simulink model "simulazionesimulinkprogetto"  (R2021a)
settings: Solver=VariableStepAuto  StartTime=0.0  StopTime=10.0  RelTol=1e-3
undefined symbols (not defined in the file): A, B, C, D
libraries: simulink x1
settings Model: Creator=micha  LastModifiedBy=micha

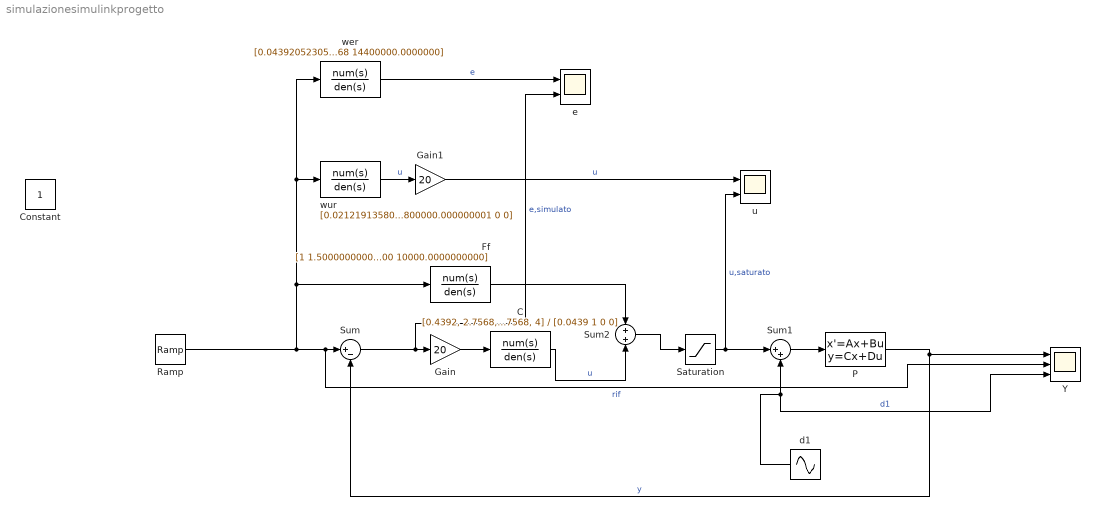
== system simulazionesimulinkprogetto ==
  C : TransferFcn  Numerator=[0.4392, 2.7568, 5.7568, 4]  Denominator=[0.0439 1 0 0]  ContinuousStateAttributes='C'
  Constant : Constant
  Ff : TransferFcn  Numerator="[1\t1.50000000000000\t18.0000000000000]"  Denominator="[1.00000000000000\t200.000000000000\t10000.0000000000]"  ContinuousStateAttributes='C'
  Gain : Gain  Gain=20
  Gain1 : Gain  Gain=20
  P : StateSpace  A=A  B=B  C=C  D=D  InitialCondition=0
  Ramp : simulink/Sources/Ramp  slope=1  start=0  InitialOutput=0
  Saturation : Saturate  UpperLimit=100
  Sum : Sum  Inputs=|+-
  Sum1 : Sum  Inputs=|++
  Sum2 : Sum
  Y : Scope  NumInputPorts=3
  d1 : Sin  Amplitude=300  Frequency=94  SampleTime=0.00001
  e : Scope  NumInputPorts=2
  u : Scope  NumInputPorts=2
  wer : TransferFcn  Numerator="[0.0439205230578942\t9.91586618075252\t670.193583897585\t12293.0976398057\t54987.4920081336\t420146.510637170\t747034.264458108\t3239676.00000001\t0\t0]"  Denominator="[0.0439205230578942\t9.91586618075252\t679.021609032222\t14119.3628990543\t156851.688085790\t1175749.03196680\t4557876.27342232\t16131532.7034383\t22212555.3203368\t14400000.0000000]"  ContinuousStateAttributes='C'
  wur : TransferFcn  Numerator="[0.0212191358024692\t4.54087420716004\t316.280144060100\t6758.67358426242\t46190.2722783823\t218931.292402326\t693679.987577993\t1142250.54261852\t720000.000000002\t0\t0]"  Denominator="[0.00192901234567901\t0.476537033770110\t38.9893226441832\t1232.08976222877\t18458.4286313574\t158625.941887430\t805742.713733091\t1202500.60290947\t800000.000000001\t0\t0]"  ContinuousStateAttributes='C'
  wires:
  Gain/1 -> C/1
  Sum/1 -> e/2, Gain/1  "e,simulato"
  d1/1 -> Sum1/2, Y/3  "d1"
  Sum1/1 -> P/1
  P/1 -> Y/1, Sum/2  "y"
  Ramp/1 -> wer/1, wur/1, Ff/1, Y/2, Sum/1  "rif"
  wur/1 -> Gain1/1  "u"
  wer/1 -> e/1  "e"
  C/1 -> Sum2/2  "u"
  Saturation/1 -> u/2, Sum1/1  "u,saturato"
  Gain1/1 -> u/1  "u"
  Ff/1 -> Sum2/1
  Sum2/1 -> Saturation/1
